simulink model "slave_model"  (R2017a)
settings: Solver=VariableStepAuto  StartTime=0.0  StopTime=10.0  MaxStep=1e-4  RelTol=1e-3
values from neighbouring files (symbols this model uses):
  adc_lsb = adc_ref/(adc_max+1)    (= 0.00118408203125)    [Slave.m]
  bal_ki = -1*bal_ki    [Slave.m]
  bal_kp = -1*bal_kp    [Slave.m]
  FIR_Coef = fir1(N,fc/(0.5*fs),'low')    [Slave.m]
  fs = 100    [Slave.m]
  Ibleed_max = 4.2/Rb    (= 0.42)    [Slave.m]
  Icharge = 300E-3    (= 0.3)    [Slave.m]
  pwm_max = 2^pwm_res-1    (= 31)    [Slave.m]
  pwm_min = 0    [Slave.m]
  Vtarget = 4.15    [Slave.m]
undefined symbols (not defined in the file or in its folder): Ion, Lithium
libraries: powerlib x3, electricdrivelib x1, simulink x1, powerlib_meascontrol x1
settings Model: Creator=christian-dsa  LastModifiedBy=christian-dsa

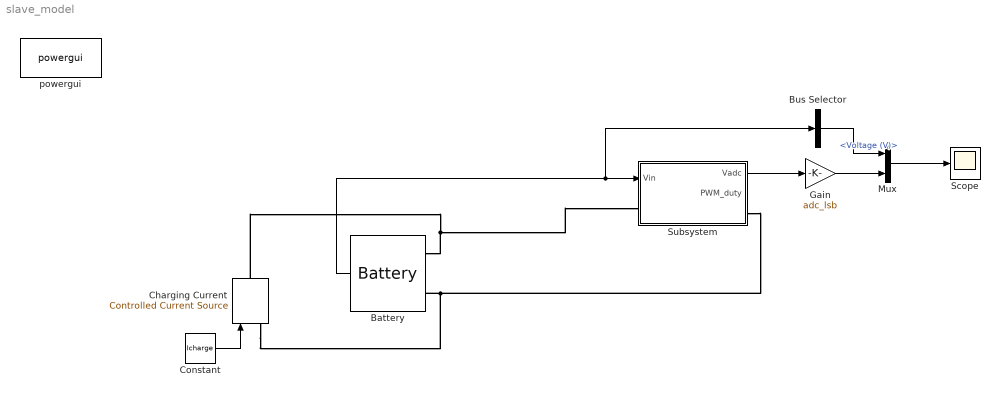
== system slave_model ==
  Battery : electricdrivelib/Extra Sources/Battery  BatType=Lithium-Ion  ShowTempParam=off  ThermalPreset=no  ShowAgeParam=off  NomV=3.6  NomQ=3  SOC=97  Batt_Tr=30  PresetModel=off  MaxQ=3  MinV=2.5  FullV=4.2  Dis_rate=2.3478  R=0.013333  Normal_OP=0.8*3  expZone="[4      0.2653]"  current=[6.5 13 32.5]  Units=Time  Tci=20  NomT=20  T2=-30  MaxQ2=4.8  FullV2=7.1  Normal_OP2=5.655  expZone2="[6.58           1]"  Rca=0.6  ti=2000  Dp=0  Neq0=0  Tsim=1e6  Ta1=25  Qeol=5.4*0.9  Reol=0.013333*1.2  Char_age=[2.3478, 3]  Dis_age=[2.3478, 10]  N1=1500  N2=10500  N3=1000  N4=1400  Ta2=45  N5=950
  Bus Selector : BusSelector  OutputSignals=Voltage (V)
  Charging Current : powerlib/Electrical Sources/Controlled Current Source  Initialize=on  Source_Type=DC  Amplitude=0  Phase=0  Frequency=0  Measurements=None
  Constant : Constant  Value=Icharge
  Gain : Gain  Gain=adc_lsb
  Mux : Mux  Inputs=2
  Scope : Scope
  Subsystem : Subsystem
  powergui : powerlib/powergui  Priority=1  SimulationMode=Continuous  SampleTime=50e-6  frequency=60  Iterations=50  frequencyindice=0  Pbase=100e6  ErrMax=1e-4  UnitsV=kV  UnitsW=MW  buscounter=0  FunctionMessages=off  echomessages=off  EnableUseOfTLC=off  CurrentSourceSwitches=off  DisableSnubberDevices=off  DisableRonSwitches=off  DisableVfSwitches=off  DisplayEquations=off  SolverType=Tustin/Backward Euler (TBE)  Interpol=off  ExternalGateDelay=off  methode=off  Ts=100  x0status=blocks  SPID=on  SwTol=0  HookPort=off  RestoreLinks=warning  ResistiveCurrentMeasurement=off  Frange=[0:2:500]  Ylog=off  Xlog=on  ShowGrid=off  save=off  variable=ZData  structure=0  ZoomFFT=off  StartTime=0.0  cycles=1  DisplayStyle=1  fundamental=60  FreqAxis=off  MaxFrequency=1000  frequencyindicesteady=1  RmsSteady=1  display=off
  wires:
  Constant/1 -> Charging Current/1
  Battery/1 -> Bus Selector/1, Subsystem/1(Vin)
  Subsystem/1(Vadc) -> Gain/1
  Gain/1 -> Mux/2
  Mux/1 -> Scope/1
  Bus Selector/1 -> Mux/1  "<Voltage (V)>"
  connections:
  Battery/LConn2 -- Charging Current/LConn1 -- Subsystem/RConn1
  Battery/LConn1 -- Subsystem/LConn1 -- Charging Current/RConn1

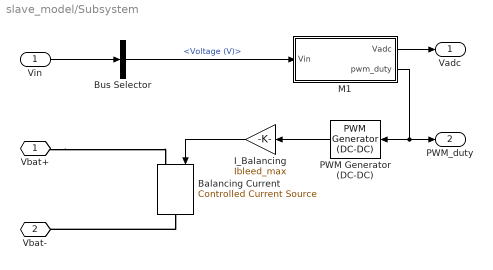
== system slave_model/Subsystem ==
  Vin : Inport
  Balancing Current : powerlib/Electrical Sources/Controlled Current Source  Initialize=on  Source_Type=DC  Amplitude=0  Phase=0  Frequency=0  Measurements=None
  Bus Selector : BusSelector  OutputSignals=Voltage (V)
  I_Balancing : Gain  Gain=Ibleed_max
  M1 : Subsystem
  PWM Generator (DC-DC) : powerlib_meascontrol/Pulse & Signal Generators/PWM Generator (DC-DC)  Fsw=1000  Ts=0
  Vbat+ : PMIOPort  Port=1  Side=Left
  Vbat- : PMIOPort  Port=2  Side=Right
  Vadc : Outport
  PWM_duty : Outport  Port=2
  wires:
  PWM Generator (DC-DC)/1 -> I_Balancing/1
  I_Balancing/1 -> Balancing Current/1
  M1/1(Vadc) -> Vadc/1
  Bus Selector/1 -> M1/1(Vin)  "<Voltage (V)>"
  M1/2(pwm_duty) -> PWM_duty/1, PWM Generator (DC-DC)/1
  Vin/1 -> Bus Selector/1
  connections:
  Balancing Current/RConn1 -- Vbat-/RConn1
  Vbat+/RConn1 -- Balancing Current/LConn1

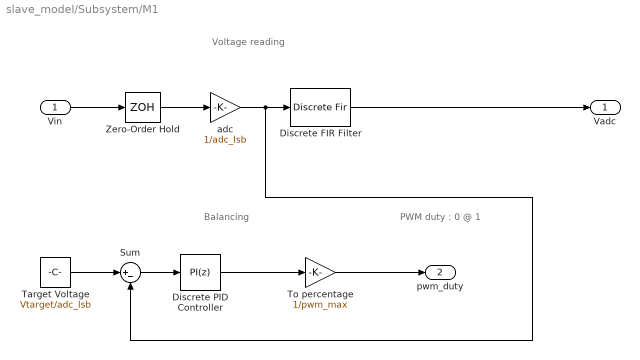
== system slave_model/Subsystem/M1 ==
  note: PWM duty : 0 @ 1
  note: Balancing
  note: Voltage reading
  Vin : Inport
  Discrete FIR Filter : DiscreteFir  Coefficients=FIR_Coef  InitialStates=4
  Discrete PID Controller : simulink/Continuous/PID Controller  Controller=PI  TimeDomain=Discrete-time  SampleTime=-1  IntegratorMethod=Forward Euler  FilterMethod=Forward Euler  Form=Parallel  UseFilter=on  ControllerParametersSource=internal  P=bal_kp  I=bal_ki  D=0  N=100  InitialConditionSource=internal  InitialConditionForIntegrator=0  InitialConditionForFilter=0  ExternalReset=none  LimitOutput=on  UpperSaturationLimit=pwm_max  LowerSaturationLimit=pwm_min  LinearizeAsGain=off  AntiWindupMode=clamping  Kb=1  TrackingMode=off  Kt=1  PParamMin=[]  PParamMax=[]  IParamMin=[]  IParamMax=[]  DParamMin=[]  DParamMax=[]  NParamMin=[]  NParamMax=[]  KbParamMin=[]  KbParamMax=[]  KtParamMin=[]  KtParamMax=[]  POutMin=[]  POutMax=[]  IOutMin=[]  IOutMax=[]  DOutMin=[]  DOutMax=[]  NOutMin=[]  NOutMax=[]  KbOutMin=[]  KbOutMax=[]  KtOutMin=[]  KtOutMax=[]  IntegratorOutMin=[]  IntegratorOutMax=[]  FilterOutMin=[]  FilterOutMax=[]  SumOutMin=[]  SumOutMax=[]  SumI1OutMin=[]  SumI1OutMax=[]  SumI2OutMin=[]  SumI2OutMax=[]  SumI3OutMin=[]  SumI3OutMax=[]  SumDOutMin=[]  SumDOutMax=[]  SaturationOutMin=[]  SaturationOutMax=[]  IntegratorContinuousStateAttributes=''  IntegratorStateMustResolveToSignalObject=off  IntegratorRTWStateStorageClass=Auto  FilterContinuousStateAttributes=''  FilterStateMustResolveToSignalObject=off  FilterRTWStateStorageClass=Auto  DifferentiatorICPrevScaledInput=0  DifferentiatorOutMin=[]  DifferentiatorOutMax=[]  InitialConditionSetting=State (most efficient)
  Sum : Sum  Inputs=|+-
  Target Voltage : Constant  Value=Vtarget/adc_lsb
  To percentage : Gain  Gain=1/pwm_max
  Zero-Order Hold : ZeroOrderHold  SampleTime=1/fs
  adc : Gain  Gain=1/adc_lsb
  Vadc : Outport
  pwm_duty : Outport  Port=2
  wires:
  Vin/1 -> Zero-Order Hold/1
  adc/1 -> Sum/2, Discrete FIR Filter/1
  Sum/1 -> Discrete PID Controller/1
  Target Voltage/1 -> Sum/1
  Discrete PID Controller/1 -> To percentage/1
  To percentage/1 -> pwm_duty/1
  Discrete FIR Filter/1 -> Vadc/1
  Zero-Order Hold/1 -> adc/1
